simulink model "Traffic"  (R2021a)
settings: Solver=FixedStepDiscrete  StartTime=0.0  StopTime=10.0  FixedStep=3  MaxStep=1  RelTol=1e-3  EnableMultiTasking=on
settings Model: Creator=elkny  LastModifiedBy=elkny
settings DataIOCC: ReturnWorkspaceOutputs=off
settings OptimizationCC: DefaultParameterBehavior=Inlined  InlineInvariantSignals=on  EnableMemcpy=off  LifeSpan=1  EfficientTunableParamExpr=on
settings DebuggingCC: UnderspecifiedInitializationDetection=Classic  MergeDetectMultiDrivingBlocksExec=none  SFMachineParentedDataDiag=warning  ArithmeticOperatorsInVariantConditions=warning
settings ModelReferenceCC: PropagateSignalLabelsOutOfModel=off
settings SFSimCC: MATLABDynamicMemAlloc=off  CustomCodeUndefinedFunction=UseInterfaceOnly
settings RTWCC: SystemTargetFile=ert.tlc  GenCodeOnly=on  TemplateMakefile=ert_default_tmf  GenerateReport=on  IncludeHyperlinkInReport=on  LaunchReport=on  GenerateTraceInfo=on  GenerateTraceReport=on  GenerateTraceReportSl=on  GenerateTraceReportSf=on  GenerateTraceReportEml=on
settings CodeAppCC: ForceParamTrailComments=on  IgnoreCustomStorageClasses=off  OperatorAnnotations=on  SimulinkDataObjDesc=on  SFDataObjDesc=on  MATLABFcnDesc=on  InsertBlockDesc=on  StateflowObjectComments=on  MATLABSourceComments=on
settings ERTTargetCC: MultiwordLength=2048  GenerateSampleERTMain=on  InlinedParameterPlacement=NonHierarchical  ERTCustomFileTemplate=example_file_process.tlc

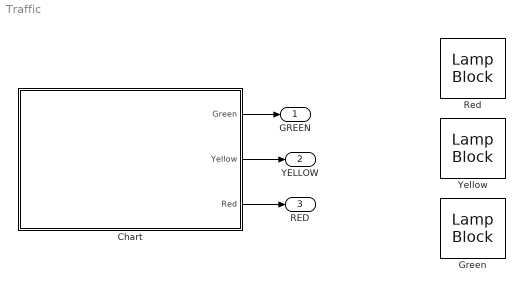
== system Traffic ==
  Chart : Stateflow chart  TreatAsAtomicUnit=on
  Green : LampBlock
  Red : LampBlock
  Yellow : LampBlock
  GREEN : Outport
  YELLOW : Outport  Port=2
  RED : Outport  Port=3
  wires:
  Chart/1(Green) -> GREEN/1
  Chart/2(Yellow) -> YELLOW/1
  Chart/3(Red) -> RED/1

== stateflow chart Traffic/Chart ==
  state Stop
    entry:
    Red=1;
    Yellow=0;
    Green=0
  state wait
    entry:
    Red=0;
    Yellow=1;
    Green=0;
  state Go
    entry:
    Red=0;
    Yellow=0;
    Green=1;
  (default) -> Stop
  Go -> Stop : after(3,sec)
  Stop -> wait : after(3,sec)
  wait -> Go : after(3,sec)
  data: Green output; Yellow output; Red output
